simulink model "Fixed_Channel_Model_12_Channels"  (R2023a)
settings: Solver=ode23tb  StartTime=0.0  StopTime=3  RelTol=1e-3
libraries: dspfdesign x13, dspsrcs4 x12, dspvision x2
settings Model: Creator=zacha  LastModifiedBy=zacha
settings DebuggingCC: UnconnectedInputMsg=warning  UnconnectedOutputMsg=warning  UnconnectedLineMsg=warning
settings ModelReferenceCC: EnableRefExpFcnMdlSchedulingChecks=on
settings RTWCC: DLArmComputeVersion=19.05

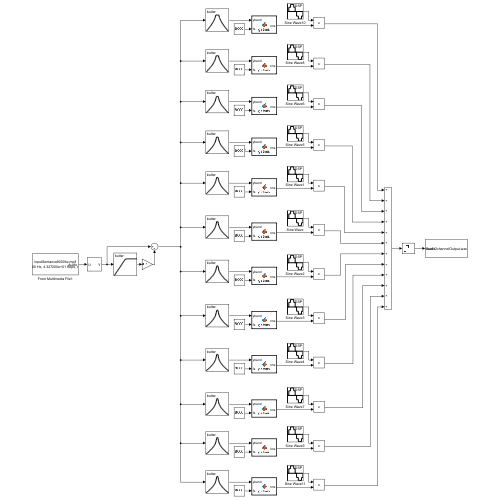
[thumbnail: Simulink's stored preview of the top-level diagram]
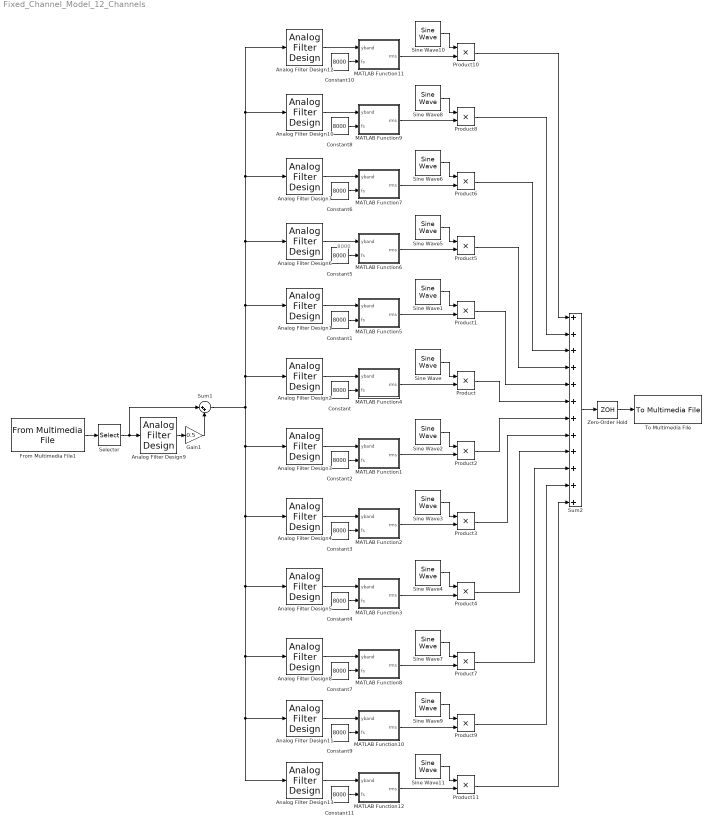
== system Fixed_Channel_Model_12_Channels ==
  note: 8000
  Analog Filter Design1 : dspfdesign/Analog Filter Design  method=Butterworth  filttype=Bandpass  N=6  Wlo=7270.731100909943  Whi=9342.20234416085  Rp=2  Rs=40
  Analog Filter Design10 : dspfdesign/Analog Filter Design  method=Butterworth  filttype=Bandpass  N=6  Wlo=2682.11608936905  Whi=3980.63717227876  Rp=2  Rs=40
  Analog Filter Design11 : dspfdesign/Analog Filter Design  method=Butterworth  filttype=Bandpass  N=6  Wlo=26268.0114433584  Whi=31539.5661213298  Rp=2  Rs=40
  Analog Filter Design12 : dspfdesign/Analog Filter Design  method=Butterworth  filttype=Bandpass  N=6  Wlo=1570.79632679490  Whi=2682.11608936905  Rp=2  Rs=40
  Analog Filter Design13 : dspfdesign/Analog Filter Design  method=Butterworth  filttype=Bandpass  N=6  Wlo=31539.5661213298  Whi=37699.1118430775  Rp=2  Rs=40
  Analog Filter Design2 : dspfdesign/Analog Filter Design  method=Butterworth  filttype=Bandpass  N=6  Wlo=9342.20234416085  Whi=11762.6119981492  Rp=2  Rs=40
  Analog Filter Design3 : dspfdesign/Analog Filter Design  method=Butterworth  filttype=Bandpass  N=6  Wlo=11762.6119981492  Whi=14590.7385831584  Rp=2  Rs=40
  Analog Filter Design4 : dspfdesign/Analog Filter Design  method=Butterworth  filttype=Bandpass  N=6  Wlo=14590.7385831584  Whi=17895.2618351030  Rp=2  Rs=40
  Analog Filter Design5 : dspfdesign/Analog Filter Design  method=Butterworth  filttype=Bandpass  N=6  Wlo=17895.2618351030  Whi=21756.4305609036  Rp=2  Rs=40
  Analog Filter Design6 : dspfdesign/Analog Filter Design  method=Butterworth  filttype=Bandpass  N=6  Wlo=5497.89355477605  Whi=7270.73110090994  Rp=2  Rs=40
  Analog Filter Design7 : dspfdesign/Analog Filter Design  method=Butterworth  filttype=Bandpass  N=6  Wlo=3980.63717227876  Whi=5497.89355477605  Rp=2  Rs=40
  Analog Filter Design8 : dspfdesign/Analog Filter Design  method=Butterworth  filttype=Bandpass  N=6  Wlo=21756.4305609036  Whi=26268.0114433584  Rp=2  Rs=40
  Analog Filter Design9 : dspfdesign/Analog Filter Design  method=Butterworth  filttype=Highpass  N=6  Wlo=7539.82236  Whi=80  Rp=2  Rs=40
  Constant{,1..11} (12 alike) : Constant  Value=8000
  From Multimedia File1 : dspvision/From Multimedia File  inputFilename=C:\Users\zacha\Desktop\Cochlear\Media\inputSentance8000hz.mp3  readRange=[1 Inf]  loop=on  numPlays=1  outputStreams=Audio only  videoDataType=single  audioDataType=double  inheritSampleTime=off  userDefinedSampleTime=1/8000  noAudioOutput=off  isIntensityVideo=off  fourcc=RGB  colorVideoFormat=Separate color signals  outputEOF=off  dataOrg=Column-major  audioFrameSize=1  computeAudioFrameSize=off  outSamplingMode=Sample based
      settings: LibrarySourceBlock=dspsrcs4/From Multimedia File
  Gain1 : Gain  Gain=0.5
  MATLAB Function1 : MATLAB Function  TreatAsAtomicUnit=on
  MATLAB Function10 : MATLAB Function  TreatAsAtomicUnit=on
  MATLAB Function11 : MATLAB Function  TreatAsAtomicUnit=on
  MATLAB Function12 : MATLAB Function  TreatAsAtomicUnit=on
  MATLAB Function2 : MATLAB Function  TreatAsAtomicUnit=on
  MATLAB Function3 : MATLAB Function  TreatAsAtomicUnit=on
  MATLAB Function4 : MATLAB Function  TreatAsAtomicUnit=on
  MATLAB Function5 : MATLAB Function  TreatAsAtomicUnit=on
  MATLAB Function6 : MATLAB Function  TreatAsAtomicUnit=on
  MATLAB Function7 : MATLAB Function  TreatAsAtomicUnit=on
  MATLAB Function8 : MATLAB Function  TreatAsAtomicUnit=on
  MATLAB Function9 : MATLAB Function  TreatAsAtomicUnit=on
  Product{,1..11} (12 alike) : Product
  Selector : Selector  NumberOfDimensions=2  InputPortWidth=3  IndexOptions=Select all,Index vector (dialog)  Indices=[2],1  OutputSizes=1,1
  Sine Wave : dspsrcs4/Sine Wave  Amplitude=1  Frequency=1679.46776280768  Phase=0  SampleMode=Discrete  OutComplex=Real  CompMethod=Trigonometric fcn  TableSize=Speed  SampleTime=1/8000  SamplesPerFrame=1  ResetState=Restart at time zero  OutputFrames=off  dataType=double  wordLen=16  udDataType=sfix(16)  fracBitsMode=Best precision  numFracBits=15  OutDataTypeStr=double  LastOutDataTypeStr=double
  Sine Wave1 : dspsrcs4/Sine Wave  Amplitude=1  Frequency=1322.01523851984  Phase=0  SampleMode=Discrete  OutComplex=Real  CompMethod=Trigonometric fcn  TableSize=Speed  SampleTime=1/8000  SamplesPerFrame=1  ResetState=Restart at time zero  OutputFrames=off  dataType=double  wordLen=16  udDataType=sfix(16)  fracBitsMode=Best precision  numFracBits=15  OutDataTypeStr=double  LastOutDataTypeStr=double
  Sine Wave10 : dspsrcs4/Sine Wave  Amplitude=1  Frequency=338.436016784694  Phase=0  SampleMode=Discrete  OutComplex=Real  CompMethod=Trigonometric fcn  TableSize=Speed  SampleTime=1/8000  SamplesPerFrame=1  ResetState=Restart at time zero  OutputFrames=off  dataType=double  wordLen=16  udDataType=sfix(16)  fracBitsMode=Best precision  numFracBits=15  OutDataTypeStr=double  LastOutDataTypeStr=double
  Sine Wave11 : dspsrcs4/Sine Wave  Amplitude=1  Frequency=5509.83892559166  Phase=0  SampleMode=Discrete  OutComplex=Real  CompMethod=Trigonometric fcn  TableSize=Speed  SampleTime=1/8000  SamplesPerFrame=1  ResetState=Restart at time zero  OutputFrames=off  dataType=double  wordLen=16  udDataType=sfix(16)  fracBitsMode=Best precision  numFracBits=15  OutDataTypeStr=double  LastOutDataTypeStr=double
  Sine Wave2 : dspsrcs4/Sine Wave  Amplitude=1  Frequency=2097.13300602438  Phase=0  SampleMode=Discrete  OutComplex=Real  CompMethod=Trigonometric fcn  TableSize=Speed  SampleTime=1/8000  SamplesPerFrame=1  ResetState=Restart at time zero  OutputFrames=off  dataType=double  wordLen=16  udDataType=sfix(16)  fracBitsMode=Best precision  numFracBits=15  OutDataTypeStr=double  LastOutDataTypeStr=double
  Sine Wave3 : dspsrcs4/Sine Wave  Amplitude=1  Frequency=2585.15377392584  Phase=0  SampleMode=Discrete  OutComplex=Real  CompMethod=Trigonometric fcn  TableSize=Speed  SampleTime=1/8000  SamplesPerFrame=1  ResetState=Restart at time zero  OutputFrames=off  dataType=double  wordLen=16  udDataType=sfix(16)  fracBitsMode=Best precision  numFracBits=15  OutDataTypeStr=double  LastOutDataTypeStr=double
  Sine Wave4 : dspsrcs4/Sine Wave  Amplitude=1  Frequency=3155.38142339188  Phase=0  SampleMode=Discrete  OutComplex=Real  CompMethod=Trigonometric fcn  TableSize=Speed  SampleTime=1/8000  SamplesPerFrame=1  ResetState=Restart at time zero  OutputFrames=off  dataType=double  wordLen=16  udDataType=sfix(16)  fracBitsMode=Best precision  numFracBits=15  OutDataTypeStr=double  LastOutDataTypeStr=double
  Sine Wave5 : dspsrcs4/Sine Wave  Amplitude=1  Frequency=1016.09486521874  Phase=0  SampleMode=Discrete  OutComplex=Real  CompMethod=Trigonometric fcn  TableSize=Speed  SampleTime=1/8000  SamplesPerFrame=1  ResetState=Restart at time zero  OutputFrames=off  dataType=double  wordLen=16  udDataType=sfix(16)  fracBitsMode=Best precision  numFracBits=15  OutDataTypeStr=double  LastOutDataTypeStr=double
  Sine Wave6 : dspsrcs4/Sine Wave  Amplitude=1  Frequency=754.277509229594  Phase=0  SampleMode=Discrete  OutComplex=Real  CompMethod=Trigonometric fcn  TableSize=Speed  SampleTime=1/8000  SamplesPerFrame=1  ResetState=Restart at time zero  OutputFrames=off  dataType=double  wordLen=16  udDataType=sfix(16)  fracBitsMode=Best precision  numFracBits=15  OutDataTypeStr=double  LastOutDataTypeStr=double
  Sine Wave7 : dspsrcs4/Sine Wave  Amplitude=1  Frequency=3821.66366710417  Phase=0  SampleMode=Discrete  OutComplex=Real  CompMethod=Trigonometric fcn  TableSize=Speed  SampleTime=1/8000  SamplesPerFrame=1  ResetState=Restart at time zero  OutputFrames=off  dataType=double  wordLen=16  udDataType=sfix(16)  fracBitsMode=Best precision  numFracBits=15  OutDataTypeStr=double  LastOutDataTypeStr=double
  Sine Wave8 : dspsrcs4/Sine Wave  Amplitude=1  Frequency=530.205058096448  Phase=0  SampleMode=Discrete  OutComplex=Real  CompMethod=Trigonometric fcn  TableSize=Speed  SampleTime=1/8000  SamplesPerFrame=1  ResetState=Restart at time zero  OutputFrames=off  dataType=double  wordLen=16  udDataType=sfix(16)  fracBitsMode=Best precision  numFracBits=15  OutDataTypeStr=double  LastOutDataTypeStr=double
  Sine Wave9 : dspsrcs4/Sine Wave  Amplitude=1  Frequency=4600.18085879414  Phase=0  SampleMode=Discrete  OutComplex=Real  CompMethod=Trigonometric fcn  TableSize=Speed  SampleTime=1/8000  SamplesPerFrame=1  ResetState=Restart at time zero  OutputFrames=off  dataType=double  wordLen=16  udDataType=sfix(16)  fracBitsMode=Best precision  numFracBits=15  OutDataTypeStr=double  LastOutDataTypeStr=double
  Sum1 : Sum  Inputs=|++
  Sum2 : Sum  Inputs=++++++++++++
  To Multimedia File : dspvision/To Multimedia File  outputFilename=C:\Users\zacha\Desktop\Cochlear\Media\fixed12channelOutput.wav  streamSelection=Audio only  videoCompressor=None (uncompressed)  audioCompressor=None (uncompressed)  imagePorts=Separate color signals  fileType=WAV  audioDatatype=16-bit integer  fourcc=RGB  videoQuality=75  mj2000CompFactor=10
      settings: LibrarySourceBlock=dspsnks4/To Multimedia File
  Zero-Order Hold : ZeroOrderHold  SampleTime=-1
  wires:
  Analog Filter Design2/1 -> MATLAB Function4/1(yband)
  Constant/1 -> MATLAB Function4/2(fs)
  MATLAB Function4/1(rms) -> Product/2
  Sine Wave/1 -> Product/1
  Sine Wave1/1 -> Product1/1
  Analog Filter Design1/1 -> MATLAB Function5/1(yband)
  MATLAB Function5/1(rms) -> Product1/2
  Constant1/1 -> MATLAB Function5/2(fs)
  Sine Wave2/1 -> Product2/1
  Analog Filter Design3/1 -> MATLAB Function1/1(yband)
  MATLAB Function1/1(rms) -> Product2/2
  Constant2/1 -> MATLAB Function1/2(fs)
  Sine Wave3/1 -> Product3/1
  MATLAB Function2/1(rms) -> Product3/2
  Analog Filter Design4/1 -> MATLAB Function2/1(yband)
  Constant3/1 -> MATLAB Function2/2(fs)
  Sine Wave4/1 -> Product4/1
  MATLAB Function3/1(rms) -> Product4/2
  Analog Filter Design5/1 -> MATLAB Function3/1(yband)
  Constant4/1 -> MATLAB Function3/2(fs)
  Sine Wave5/1 -> Product5/1
  MATLAB Function6/1(rms) -> Product5/2
  Analog Filter Design6/1 -> MATLAB Function6/1(yband)
  Constant5/1 -> MATLAB Function6/2(fs)
  Product/1 -> Sum2/6
  Product2/1 -> Sum2/7
  Product1/1 -> Sum2/5
  Product5/1 -> Sum2/4
  Product3/1 -> Sum2/8
  Product4/1 -> Sum2/9
  Constant6/1 -> MATLAB Function7/2(fs)
  MATLAB Function7/1(rms) -> Product6/2
  Analog Filter Design7/1 -> MATLAB Function7/1(yband)
  Sine Wave6/1 -> Product6/1
  Product6/1 -> Sum2/3
  Constant7/1 -> MATLAB Function8/2(fs)
  MATLAB Function8/1(rms) -> Product7/2
  Analog Filter Design8/1 -> MATLAB Function8/1(yband)
  Sine Wave7/1 -> Product7/1
  Product7/1 -> Sum2/10
  Gain1/1 -> Sum1/2
  Selector/1 -> Analog Filter Design9/1, Sum1/1
  From Multimedia File1/1 -> Selector/1
  Analog Filter Design9/1 -> Gain1/1
  MATLAB Function9/1(rms) -> Product8/2
  Analog Filter Design10/1 -> MATLAB Function9/1(yband)
  Product8/1 -> Sum2/2
  Sine Wave8/1 -> Product8/1
  Constant8/1 -> MATLAB Function9/2(fs)
  MATLAB Function10/1(rms) -> Product9/2
  Analog Filter Design11/1 -> MATLAB Function10/1(yband)
  Sine Wave9/1 -> Product9/1
  Constant9/1 -> MATLAB Function10/2(fs)
  Product9/1 -> Sum2/11
  Sum2/1 -> Zero-Order Hold/1
  Zero-Order Hold/1 -> To Multimedia File/1
  Constant10/1 -> MATLAB Function11/2(fs)
  Sine Wave10/1 -> Product10/1
  Analog Filter Design12/1 -> MATLAB Function11/1(yband)
  MATLAB Function11/1(rms) -> Product10/2
  Sine Wave11/1 -> Product11/1
  Analog Filter Design13/1 -> MATLAB Function12/1(yband)
  MATLAB Function12/1(rms) -> Product11/2
  Constant11/1 -> MATLAB Function12/2(fs)
  Sum1/1 -> Analog Filter Design12/1, Analog Filter Design10/1, Analog Filter Design7/1, Analog Filter Design6/1, Analog Filter Design1/1, Analog Filter Design2/1, Analog Filter Design13/1, Analog Filter Design11/1, Analog Filter Design8/1, Analog Filter Design5/1, Analog Filter Design4/1, Analog Filter Design3/1
  Product11/1 -> Sum2/12
  Product10/1 -> Sum2/1

== matlab function Fixed_Channel_Model_12_Channels/MATLAB Function2 ==
  data: yband input; rms output; fs input
function rms = getrms(yband,fs)

    y = abs(yband); %rectifying it makes it sound bad

    [b,a] = butter(2,400/(fs/2));

    z = filter(b,a,y); %this filter also makes it sound bad

    windowsize = round(4/(1000/fs)); %rms computed every 4ms = windowsize samples

    [yupper,ylower] = envelope(yband,windowsize,'rms'); %changed to yband here

    %envelope(z,windowsize,'rms');

    rms = yupper;
end

== matlab function Fixed_Channel_Model_12_Channels/MATLAB Function3 ==
  data: yband input; rms output; fs input
function rms = getrms(yband,fs)

    y = abs(yband); %rectifying it makes it sound bad

    [b,a] = butter(2,400/(fs/2));

    z = filter(b,a,y); %this filter also makes it sound bad

    windowsize = round(4/(1000/fs)); %rms computed every 4ms = windowsize samples

    [yupper,ylower] = envelope(yband,windowsize,'rms'); %changed to yband here

    %envelope(z,windowsize,'rms');

    rms = yupper;
end

== matlab function Fixed_Channel_Model_12_Channels/MATLAB Function6 ==
  data: yband input; rms output; fs input
function rms = getrms(yband,fs)

    y = abs(yband); %rectifying it makes it sound bad

    [b,a] = butter(2,400/(fs/2));

    z = filter(b,a,y); %this filter also makes it sound bad

    windowsize = round(4/(1000/fs)); %rms computed every 4ms = windowsize samples

    [yupper,ylower] = envelope(yband,windowsize,'rms'); %changed to yband here

    %envelope(z,windowsize,'rms');

    rms = yupper;
end

== matlab function Fixed_Channel_Model_12_Channels/MATLAB Function4 ==
  data: yband input; rms output; fs input
function rms = getrms(yband,fs)

    y = abs(yband); %rectifying it makes it sound bad

    [b,a] = butter(2,400/(fs/2));

    z = filter(b,a,y); %this filter also makes it sound bad

    windowsize = round(4/(1000/fs)); %rms computed every 4ms = windowsize samples

    [yupper,ylower] = envelope(yband,windowsize,'rms'); %changed to yband here

    %envelope(z,windowsize,'rms');

    rms = yupper;
end

== matlab function Fixed_Channel_Model_12_Channels/MATLAB Function5 ==
  data: yband input; rms output; fs input
function rms = getrms(yband,fs)

    y = abs(yband); %rectifying it makes it sound bad

    [b,a] = butter(2,400/(fs/2));

    z = filter(b,a,y); %this filter also makes it sound bad

    windowsize = round(4/(1000/fs)); %rms computed every 4ms = windowsize samples

    [yupper,ylower] = envelope(yband,windowsize,'rms'); %changed to yband here

    %envelope(z,windowsize,'rms');

    rms = yupper;
end

== matlab function Fixed_Channel_Model_12_Channels/MATLAB Function7 ==
  data: yband input; rms output; fs input
function rms = getrms(yband,fs)

    y = abs(yband); %rectifying it makes it sound bad

    [b,a] = butter(2,400/(fs/2));

    z = filter(b,a,y); %this filter also makes it sound bad

    windowsize = round(4/(1000/fs)); %rms computed every 4ms = windowsize samples

    [yupper,ylower] = envelope(yband,windowsize,'rms'); %changed to yband here

    %envelope(z,windowsize,'rms');

    rms = yupper;
end

== matlab function Fixed_Channel_Model_12_Channels/MATLAB Function8 ==
  data: yband input; rms output; fs input
function rms = getrms(yband,fs)

    y = abs(yband); %rectifying it makes it sound bad

    [b,a] = butter(2,400/(fs/2));

    z = filter(b,a,y); %this filter also makes it sound bad

    windowsize = round(4/(1000/fs)); %rms computed every 4ms = windowsize samples

    [yupper,ylower] = envelope(yband,windowsize,'rms'); %changed to yband here

    %envelope(z,windowsize,'rms');

    rms = yupper;
end

== matlab function Fixed_Channel_Model_12_Channels/MATLAB Function9 ==
  data: yband input; rms output; fs input
function rms = getrms(yband,fs)

    y = abs(yband); %rectifying it makes it sound bad

    [b,a] = butter(2,400/(fs/2));

    z = filter(b,a,y); %this filter also makes it sound bad

    windowsize = round(4/(1000/fs)); %rms computed every 4ms = windowsize samples

    [yupper,ylower] = envelope(yband,windowsize,'rms'); %changed to yband here

    %envelope(z,windowsize,'rms');

    rms = yupper;
end

== matlab function Fixed_Channel_Model_12_Channels/MATLAB Function10 ==
  data: yband input; rms output; fs input
function rms = getrms(yband,fs)

    y = abs(yband); %rectifying it makes it sound bad

    [b,a] = butter(2,400/(fs/2));

    z = filter(b,a,y); %this filter also makes it sound bad

    windowsize = round(4/(1000/fs)); %rms computed every 4ms = windowsize samples

    [yupper,ylower] = envelope(yband,windowsize,'rms'); %changed to yband here

    %envelope(z,windowsize,'rms');

    rms = yupper;
end

== matlab function Fixed_Channel_Model_12_Channels/MATLAB Function11 ==
  data: yband input; rms output; fs input
function rms = getrms(yband,fs)

    y = abs(yband); %rectifying it makes it sound bad

    [b,a] = butter(2,400/(fs/2));

    z = filter(b,a,y); %this filter also makes it sound bad

    windowsize = round(4/(1000/fs)); %rms computed every 4ms = windowsize samples

    [yupper,ylower] = envelope(yband,windowsize,'rms'); %changed to yband here

    %envelope(z,windowsize,'rms');

    rms = yupper;
end

== matlab function Fixed_Channel_Model_12_Channels/MATLAB Function1 ==
  data: yband input; rms output; fs input
function rms = getrms(yband,fs)

    y = abs(yband); %rectifying it makes it sound bad

    [b,a] = butter(2,400/(fs/2));

    z = filter(b,a,y); %this filter also makes it sound bad

    windowsize = round(4/(1000/fs)); %rms computed every 4ms = windowsize samples

    [yupper,ylower] = envelope(yband,windowsize,'rms'); %changed to yband here

    %envelope(z,windowsize,'rms');

    rms = yupper;
end

== matlab function Fixed_Channel_Model_12_Channels/MATLAB Function12 ==
  data: yband input; rms output; fs input
function rms = getrms(yband,fs)

    y = abs(yband); %rectifying it makes it sound bad

    [b,a] = butter(2,400/(fs/2));

    z = filter(b,a,y); %this filter also makes it sound bad

    windowsize = round(4/(1000/fs)); %rms computed every 4ms = windowsize samples

    [yupper,ylower] = envelope(yband,windowsize,'rms'); %changed to yband here

    %envelope(z,windowsize,'rms');

    rms = yupper;
end
